simulink model "sampleModel43"  (R2021b)
settings: Solver=VariableStepAuto  StartTime=0.0  StopTime=10.0  RelTol=1e-3
undefined symbols (not defined in the file or in its folder): magnitude
libraries: simulink x5
settings Model: Creator=user  LastModifiedBy=user

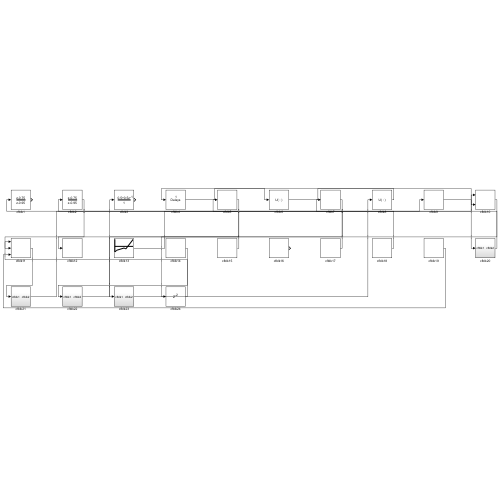
[thumbnail: Simulink's stored preview of the top-level diagram]
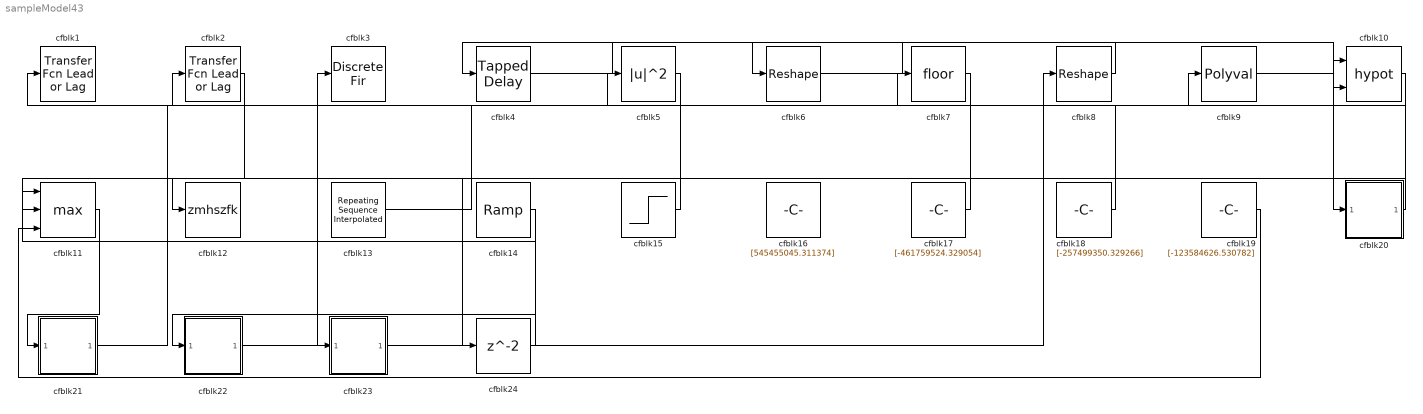
== system sampleModel43 ==
  cfblk1 : simulink/Discrete/Transfer Fcn Lead or Lag  PoleZ=0.95  ZeroZ=0.75  ICPrevOutput=0.0  ICPrevInput=0.0  DoSatur=off
      settings: SourceProductBaseCode=SL
  cfblk10 : Math  Operator=hypot  SaturateOnIntegerOverflow=on
  cfblk11 : MinMax  Function=max  Inputs=3
  cfblk12 : ToWorkspace  VariableName=zmhszfk  SaveFormat=Timeseries  SampleTime=-1
  cfblk13 : simulink/Sources/Repeating Sequence Interpolated  OutValues=[-675984985.743648, -500556045.784337, -212584635.484413, -319666678.716128, 857049767.335375]  TimeValues=[0 0.1 0.5 0.6 1].'  LookUpMeth=Use Input Nearest  tsamp=0.01  OutMin=[]  OutMax=[]  OutDataTypeStr=double  OutputDataTypeScalingMode=double  OutDataType=fixdt(0,8)  OutScaling=2^-10
  cfblk14 : simulink/Sources/Ramp  slope=[531.331533]  start=[25.556552]  InitialOutput=[620652.762937]
  cfblk15 : Step  Time=[40.000000]  Before=[-764358335.378188]  After=[236700457.841213]  SampleTime=0
  cfblk16 : Constant  Value=[545455045.311374]  SampleTime=1
  cfblk17 : Constant  Value=[-461759524.329054]  SampleTime=1
  cfblk18 : Constant  Value=[-257499350.329266]  SampleTime=1
  cfblk19 : Constant  Value=[-123584626.530782]  SampleTime=1
  cfblk2 : simulink/Discrete/Transfer Fcn Lead or Lag  PoleZ=0.95  ZeroZ=0.75  ICPrevOutput=0.0  ICPrevInput=0.0  DoSatur=off
      settings: SourceProductBaseCode=SL
  cfblk20 : Subsystem
  cfblk21 : Subsystem
  cfblk22 : Subsystem
  cfblk23 : Subsystem
  cfblk24 : Delay  SampleTime=1
  cfblk3 : DiscreteFir  SampleTime=1
  cfblk4 : simulink/Discrete/Tapped Delay  vinit=0.0  samptime=-1  NumDelays=1  DelayOrder=Oldest  includeCurrent=off
  cfblk5 : Math  Operator=magnitude^2  SaturateOnIntegerOverflow=on
  cfblk6 : Reshape
  cfblk7 : Rounding
  cfblk8 : Reshape
  cfblk9 : Polyval  Coefs=[ +2.081618890e-019, -1.441693666e-014, +4.719686976e-010, -8.536869453e-006, +1.621573104e-001, -8.087801117e+001 ]
  wires:
  cfblk4/1 -> cfblk6/1
  cfblk13/1 -> cfblk9/1
  cfblk14/1 -> cfblk22/1(cfblk1)
  cfblk22/1(cfblk2) -> cfblk3/1
  cfblk6/1 -> cfblk20/1(cfblk1)
  cfblk11/1 -> cfblk21/1(cfblk1)
  cfblk15/1 -> cfblk1/1
  cfblk17/1 -> cfblk5/1
  cfblk7/1 -> cfblk23/1(cfblk1)
  cfblk20/1(cfblk2) -> cfblk2/1
  cfblk18/1 -> cfblk7/1
  cfblk21/1(cfblk2) -> cfblk10/1
  cfblk5/1 -> cfblk11/2
  cfblk9/1 -> cfblk10/2
  cfblk19/1 -> cfblk11/3
  cfblk2/1 -> cfblk12/1
  cfblk8/1 -> cfblk4/1
  cfblk23/1(cfblk2) -> cfblk8/1
  cfblk10/1 -> cfblk24/1
  cfblk24/1 -> cfblk11/1

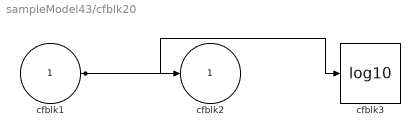
== system sampleModel43/cfblk20 ==
  cfblk1 : Inport
  cfblk3 : Math  Operator=log10  SaturateOnIntegerOverflow=on
  cfblk2 : Outport
  wires:
  cfblk1/1 -> cfblk2/1, cfblk3/1

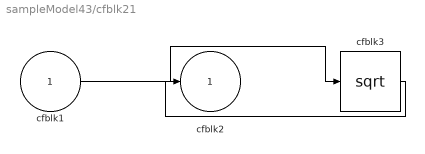
== system sampleModel43/cfblk21 ==
  cfblk1 : Inport
  cfblk3 : Sqrt  SaturateOnIntegerOverflow=on
  cfblk2 : Outport
  wires:
  cfblk1/1 -> cfblk3/1
  cfblk3/1 -> cfblk2/1

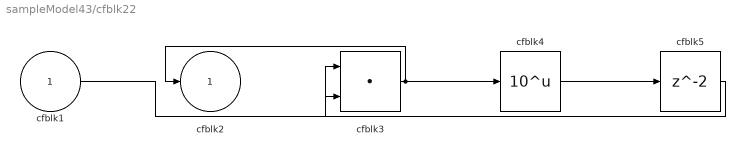
== system sampleModel43/cfblk22 ==
  cfblk1 : Inport
  cfblk3 : DotProduct  InputSameDT=on  OutDataTypeStr=Inherit: Inherit via internal rule
  cfblk4 : Math  Operator=10^u  SaturateOnIntegerOverflow=on
  cfblk5 : Delay  SampleTime=1
  cfblk2 : Outport
  wires:
  cfblk3/1 -> cfblk2/1, cfblk4/1
  cfblk1/1 -> cfblk3/1
  cfblk4/1 -> cfblk5/1
  cfblk5/1 -> cfblk3/2

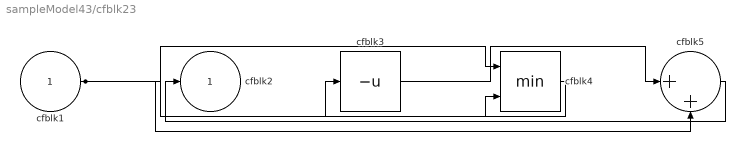
== system sampleModel43/cfblk23 ==
  cfblk1 : Inport
  cfblk3 : UnaryMinus
  cfblk4 : MinMax  Inputs=2
  cfblk5 : Sum  Inputs=|++
  cfblk2 : Outport
  wires:
  cfblk3/1 -> cfblk5/1
  cfblk5/1 -> cfblk2/1
  cfblk4/1 -> cfblk3/1
  cfblk1/1 -> cfblk5/2, cfblk4/1, cfblk4/2
